simulink model "quadri_instable"  (R2015a)
settings: Solver=ode45  StartTime=0.0  StopTime=10.0  RelTol=1e-3
values from neighbouring files (symbols this model uses):
  b = 4.83e-6    (= 4.83e-06)    [Donnees_quadri.m]
  d = 2.39e-8    (= 2.39e-08)    [Donnees_quadri.m]
  Irotor = 6*10^-6    (= 6e-06)    [Donnees_quadri.m]
  Ix = 6.22e-2    (= 0.0622)    [Donnees_quadri.m]
  Iy = 7.33e-2    (= 0.0733)    [Donnees_quadri.m]
  Iz = 9.64e-2    (= 0.0964)    [Donnees_quadri.m]
  L = 1    [Donnees_quadri.m]
settings Model: Creator=Lenovo  LastModifiedBy=Lenovo

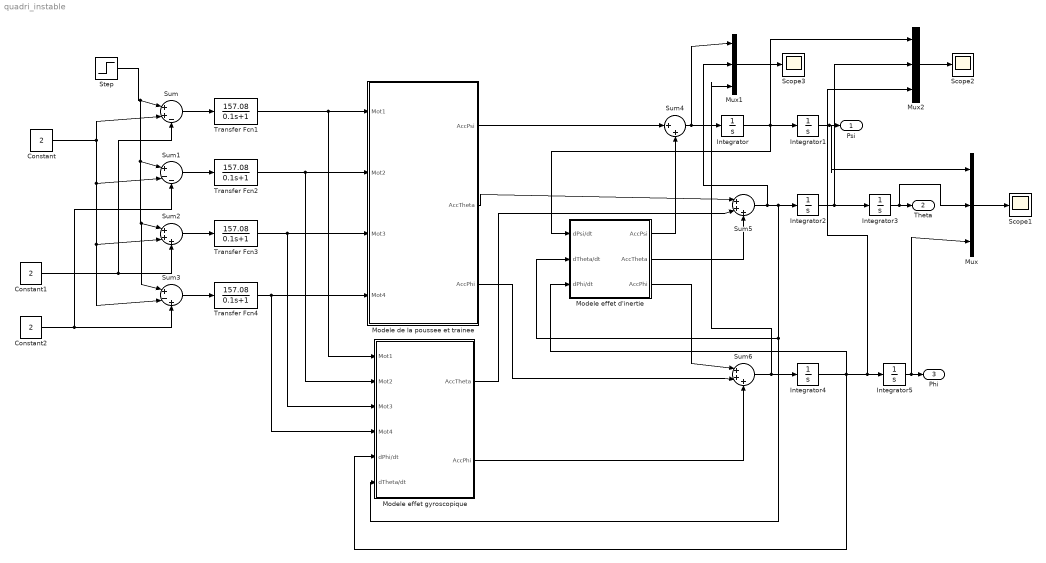
== system quadri_instable ==
  Constant : Constant  Value=2
  Constant1 : Constant  Value=2
  Constant2 : Constant  Value=2
  Integrator{,1..5} (6 alike) : Integrator
  Modele de la poussee et trainee : Subsystem
  Modele effet d'inertie : Subsystem
  Modele effet gyroscopique : Subsystem
  Mux : Mux  Inputs=3
  Mux1 : Mux  Inputs=3
  Mux2 : Mux  Inputs=3
  Scope1 : Scope
  Scope2 : Scope
  Scope3 : Scope
      settings: SaveName=ScopeData3
  Step : Step  SampleTime=0
  Sum : Sum  Inputs=|++-
  Sum1 : Sum  Inputs=|+--
  Sum2 : Sum  Inputs=|+++
  Sum3 : Sum  Inputs=|+-+
  Sum4 : Sum  Inputs=|++
  Sum5 : Sum  Inputs=|+++
  Sum6 : Sum  Inputs=|+++
  Transfer Fcn{1..4} (4 alike) : TransferFcn  Numerator=[157.08]  Denominator=[0.1 1]
  Psi : Outport
  Theta : Outport  Port=2
  Phi : Outport  Port=3
  wires:
  Sum3/1 -> Transfer Fcn4/1
  Sum2/1 -> Transfer Fcn3/1
  Sum1/1 -> Transfer Fcn2/1
  Sum/1 -> Transfer Fcn1/1
  Transfer Fcn1/1 -> Modele effet gyroscopique/1(Mot1), Modele de la poussee et trainee/1(Mot1)
  Transfer Fcn3/1 -> Modele effet gyroscopique/3(Mot3), Modele de la poussee et trainee/3(Mot3)
  Transfer Fcn4/1 -> Modele effet gyroscopique/4(Mot4), Modele de la poussee et trainee/4(Mot4)
  Transfer Fcn2/1 -> Modele effet gyroscopique/2(Mot2), Modele de la poussee et trainee/2(Mot2)
  Modele de la poussee et trainee/1(AccPsi) -> Sum4/1
  Modele de la poussee et trainee/2(AccTheta) -> Sum5/1
  Sum4/1 -> Mux1/1, Integrator/1
  Integrator2/1 -> Mux2/2, Integrator3/1
  Integrator/1 -> Mux2/1, Integrator1/1, Modele effet d'inertie/1(dPsi/dt)
  Modele effet d'inertie/3(AccPhi) -> Sum6/1
  Modele effet gyroscopique/2(AccPhi) -> Sum6/3
  Modele de la poussee et trainee/3(AccPhi) -> Sum6/2
  Modele effet d'inertie/2(AccTheta) -> Sum5/3
  Modele effet gyroscopique/1(AccTheta) -> Sum5/2
  Modele effet d'inertie/1(AccPsi) -> Sum4/2
  Integrator4/1 -> Modele effet gyroscopique/5(dPhi/dt), Modele effet d'inertie/3(dPhi/dt), Mux2/3, Integrator5/1
  Integrator5/1 -> Mux/3, Phi/1
  Integrator1/1 -> Mux/1, Psi/1
  Mux/1 -> Scope1/1
  Integrator3/1 -> Mux/2, Theta/1
  Mux2/1 -> Scope2/1
  Mux1/1 -> Scope3/1
  Sum5/1 -> Mux1/2, Modele effet gyroscopique/6(dTheta/dt), Modele effet d'inertie/2(dTheta/dt), Integrator2/1
  Sum6/1 -> Mux1/3, Integrator4/1
  Step/1 -> Sum3/1, Sum2/1, Sum1/1, Sum/1
  Constant/1 -> Sum3/2, Sum2/2, Sum1/2, Sum/2
  Constant1/1 -> Sum/3, Sum2/3
  Constant2/1 -> Sum1/3, Sum3/3

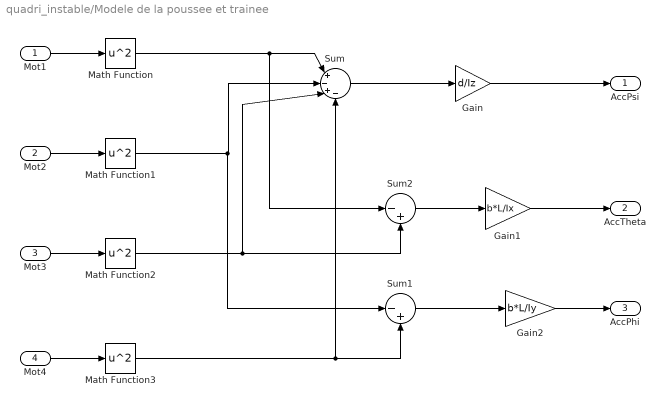
== system quadri_instable/Modele de la poussee et trainee ==
  Mot1 : Inport
  Mot2 : Inport  Port=2
  Mot3 : Inport  Port=3
  Mot4 : Inport  Port=4
  Gain : Gain  Gain=d/Iz
  Gain1 : Gain  Gain=b*L/Ix
  Gain2 : Gain  Gain=b*L/Iy
  Math Function{,1..3} (4 alike) : Math  Operator=square  SaturateOnIntegerOverflow=on
  Sum : Sum  Inputs=|+-+-
  Sum1 : Sum  Inputs=|-+
  Sum2 : Sum  Inputs=|-+
  AccPsi : Outport
  AccTheta : Outport  Port=2
  AccPhi : Outport  Port=3
  wires:
  Mot1/1 -> Math Function/1
  Mot2/1 -> Math Function1/1
  Mot3/1 -> Math Function2/1
  Mot4/1 -> Math Function3/1
  Math Function/1 -> Sum2/1, Sum/1
  Math Function1/1 -> Sum1/1, Sum/2
  Math Function2/1 -> Sum2/2, Sum/3
  Math Function3/1 -> Sum1/2, Sum/4
  Sum/1 -> Gain/1
  Gain/1 -> AccPsi/1
  Sum2/1 -> Gain1/1
  Gain1/1 -> AccTheta/1
  Gain2/1 -> AccPhi/1
  Sum1/1 -> Gain2/1

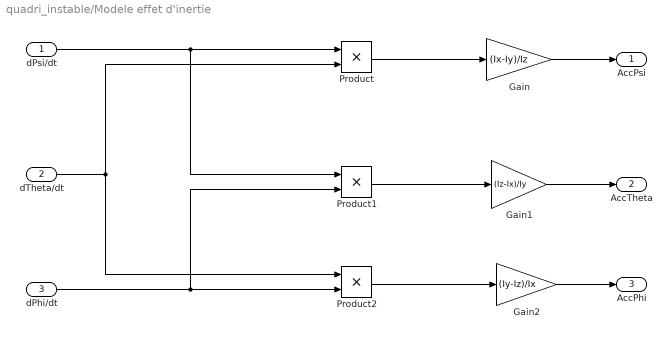
== system quadri_instable/Modele effet d'inertie ==
  dPsi/dt : Inport
  dTheta/dt : Inport  Port=2
  dPhi/dt : Inport  Port=3
  Gain : Gain  Gain=(Ix-Iy)/Iz
  Gain1 : Gain  Gain=(Iz-Ix)/Iy
  Gain2 : Gain  Gain=(Iy-Iz)/Ix
  Product : Product
  Product1 : Product
  Product2 : Product
  AccPsi : Outport
  AccTheta : Outport  Port=2
  AccPhi : Outport  Port=3
  wires:
  dPsi/dt/1 -> Product1/1, Product/1
  dPhi/dt/1 -> Product1/2, Product2/2
  Gain/1 -> AccPsi/1
  Product1/1 -> Gain1/1
  Gain1/1 -> AccTheta/1
  Gain2/1 -> AccPhi/1
  Product2/1 -> Gain2/1
  Product/1 -> Gain/1
  dTheta/dt/1 -> Product2/1, Product/2

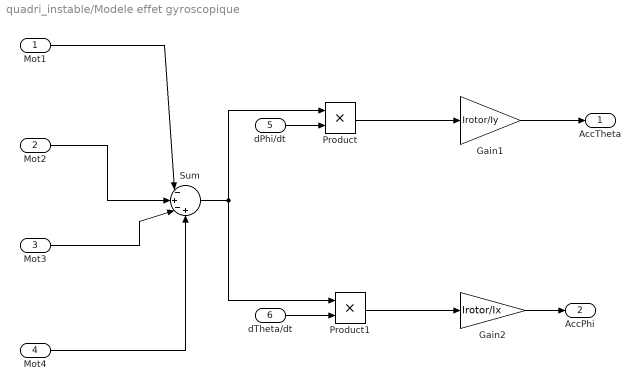
== system quadri_instable/Modele effet gyroscopique ==
  Mot1 : Inport
  Mot2 : Inport  Port=2
  Mot3 : Inport  Port=3
  Mot4 : Inport  Port=4
  dPhi/dt : Inport  Port=5
  dTheta/dt : Inport  Port=6
  Gain1 : Gain  Gain=Irotor/Iy
  Gain2 : Gain  Gain=Irotor/Ix
  Product : Product
  Product1 : Product
  Sum : Sum  Inputs=|-+-+
  AccTheta : Outport
  AccPhi : Outport  Port=2
  wires:
  Gain1/1 -> AccTheta/1
  Gain2/1 -> AccPhi/1
  Product1/1 -> Gain2/1
  Product/1 -> Gain1/1
  dPhi/dt/1 -> Product/2
  dTheta/dt/1 -> Product1/2
  Sum/1 -> Product/1, Product1/1
  Mot1/1 -> Sum/1
  Mot2/1 -> Sum/2
  Mot3/1 -> Sum/3
  Mot4/1 -> Sum/4
